simulink model "reverb_simulink"  (R2021b)
settings: Solver=VariableStepAuto  StartTime=0.0  StopTime=10.0  RelTol=1e-3
libraries: dspvision x2
settings Model: Creator=busselommers  LastModifiedBy=busselommers

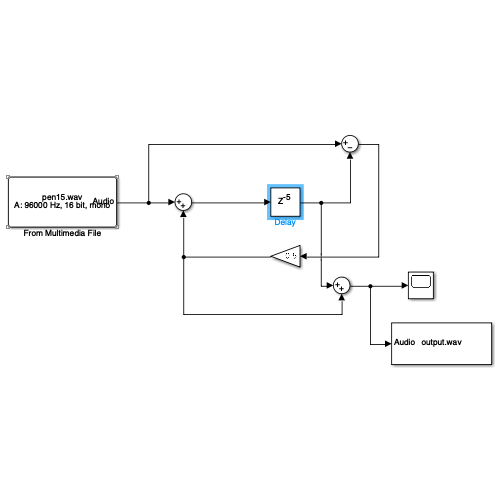
[thumbnail: Simulink's stored preview of the top-level diagram]
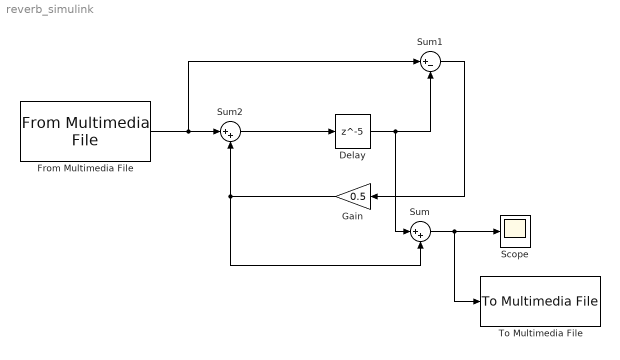
== system reverb_simulink ==
  Delay : Delay  DelayLength=5  InitialCondition=0
  From Multimedia File : dspvision/From Multimedia File  inputFilename=/Users/busselommers/Downloads/pen15.wav  readRange=[1 Inf]  loop=on  numPlays=inf  outputStreams=Audio only  videoDataType=single  audioDataType=double  inheritSampleTime=on  userDefinedSampleTime=1/30  noAudioOutput=off  isIntensityVideo=off  fourcc=RGB  colorVideoFormat=Separate color signals  outputEOF=off  dataOrg=Column-major  audioFrameSize=1024  computeAudioFrameSize=off  outSamplingMode=Sample based
  Gain : Gain  Gain=0.5
  Scope : Scope
  Sum : Sum  Inputs=|++
  Sum1 : Sum  Inputs=|+-
  Sum2 : Sum  Inputs=|++
  To Multimedia File : dspvision/To Multimedia File  outputFilename=output.wav  streamSelection=Audio only  videoCompressor=None (uncompressed)  audioCompressor=None (uncompressed)  imagePorts=Separate color signals  fileType=WAV  audioDatatype=16-bit integer  fourcc=RGB  videoQuality=75  mj2000CompFactor=10
  wires:
  From Multimedia File/1 -> Sum1/1, Sum2/1
  Sum2/1 -> Delay/1
  Delay/1 -> Sum/1, Sum1/2
  Sum1/1 -> Gain/1
  Gain/1 -> Sum/2, Sum2/2
  Sum/1 -> To Multimedia File/1, Scope/1
